simulink model "INDUCTION_ANALYSIS"  (R2022b)
settings: Solver=VariableStepAuto  StartTime=0.0  StopTime=0.5  RelTol=1e-3
libraries: simulink_extras x3, spsAsynchronousMachinepuUnitsLib x1, spsGroundLib x1, spsThreePhaseProgrammableVoltageSourceLib x1, spsThreePhaseVIMeasurementLib x1, spsThreePhaseBreakerLib x1, spsThreePhaseFaultLib x1, sps_lib x1
settings Model: Creator=ADA  LastModifiedBy=ADA
settings DebuggingCC: ParameterOverflowMsg=none  ParameterUnderflowMsg=error

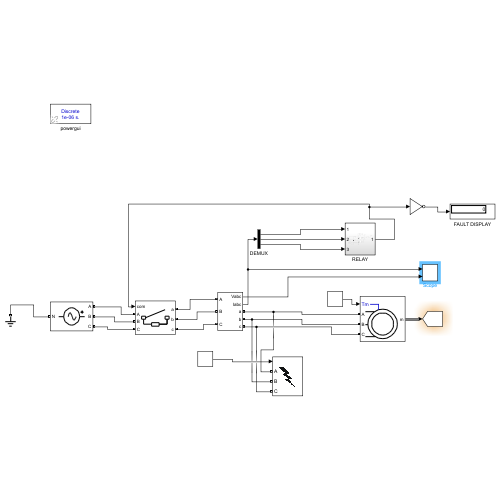
[thumbnail: Simulink's stored preview of the top-level diagram]
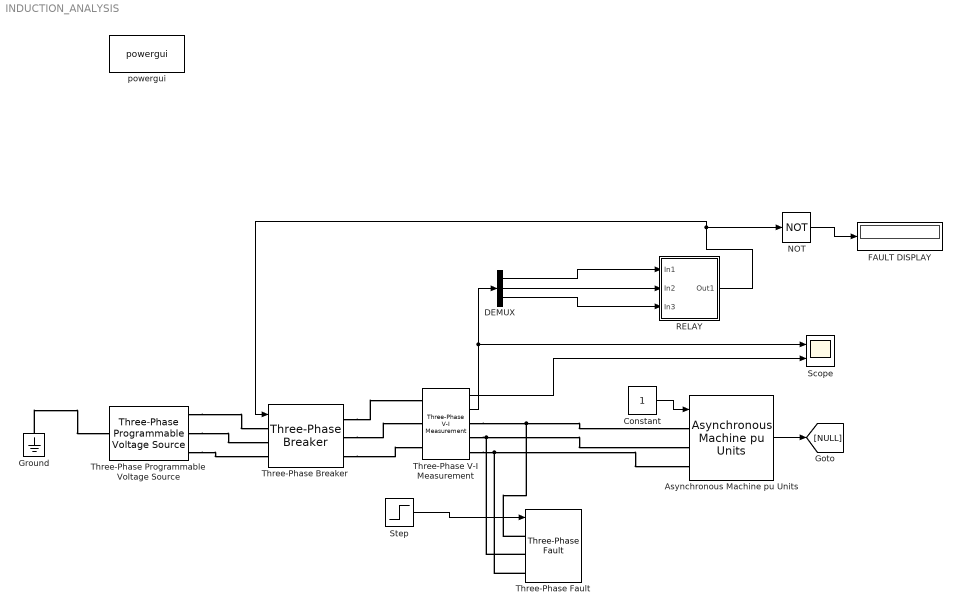
== system INDUCTION_ANALYSIS ==
  Asynchronous Machine pu Units : spsAsynchronousMachinepuUnitsLib/Asynchronous Machine pu Units  RotorType=Squirrel-cage  PresetModel=No  MechanicalLoad=Torque Tm  ShowDetailedParameters=on  ReferenceFrame=Rotor  Units=pu  MeasurementBus=off  NominalParameters=[3730 460 60]  VoltageRatio=1  Stator=[0.01965 0.0397]  Rotor=[0.01909 0.0397]  Cage1=[0.01909 0.0397]  Cage2=[0.01909 0.0397]  Lm=1.354  Mechanical=[0.09526 0.05479 2]  PolePairs=2  InitialConditions="[ 1,0   0,0,0   0,0,0 ]"  SimulateSaturation=off  Saturation="[0.212,0.4201,0.8125,1.0979,1.4799,2.2457,3.2586,4.5763,6.4763 ;   0.5,0.7,0.9,1,1.1,1.2 ,1.3,1.4,1.5]"  LoadFlowParameters=0  TsPowergui=0  TsBlock=-1  IterativeModel=Trapezoidal non iterative  IterativeDiscreteModel=Trapezoidal non iterative  Pmec=0
      settings: LibrarySourceBlock=|
      | sps_lib/Electrical Machines/Asynchronous Machine
      | pu Units
  Constant : Constant
  DEMUX : Demux  Outputs=3
  FAULT DISPLAY : Display
  Ground : spsGroundLib/Ground  LConnTagsString=a
  NOT : Logic  Operator=NOT  IconShape=distinctive  AllPortsSameDT=off  OutDataTypeStr=boolean
  RELAY : Subsystem
  Scope : Scope  NumInputPorts=2
  Step : Step  SampleTime=0
  Three-Phase Programmable Voltage Source : spsThreePhaseProgrammableVoltageSourceLib/Three-Phase Programmable Voltage Source  PositiveSequence="[100  0 50]"  VariationEntity=None  VariationType=Table of time-amplitude pairs  VariationTypeAlt=Step  VariationStep=0.5  VariationRate=10  VariationMagnitude=0.3  VariationFrequency=2  VariationTiming=[1 2]  VariationPhaseA=off  Amplitudes=[1 0.8 1.2 1.0]  TimeValues=[0 0.1 0.15 0.2]  HarmonicGeneration=off  HarmonicA=[3 0.2 -25 0]  HarmonicB=[2 0.15 35 2]  Timing="[0.05  3]"  BusType=swing  Pref=0  Qref=0  Qmin=-inf  Qmax=inf
  Three-Phase V-I Measurement : spsThreePhaseVIMeasurementLib/Three-Phase V-I Measurement  VoltageMeasurement=phase-to-ground  SetLabelV=off  LabelV=Vabc  Vpu=off  VpuLL=off  CurrentMeasurement=yes  SetLabelI=off  LabelI=Iabc  Ipu=off  Pbase=100e6  Vbase=500e3  OutputType=Complex  PhasorSimulation=off  PSBequivalent=0
  Three-Phase Breaker : spsThreePhaseBreakerLib/Three-Phase Breaker  InitialState=open  SwitchA=on  SwitchB=on  SwitchC=on  SwitchTimes="[1/60  5/60]"  External=on  BreakerResistance=0.01  SnubberResistance=1e6  SnubberCapacitance=inf  Measurements=None
  Three-Phase Fault : spsThreePhaseFaultLib/Three-Phase Fault  InitialStates=0  FaultA=on  FaultB=on  FaultC=on  GroundFault=on  SwitchTimes="[1/60  5/60]"  External=on  SwitchStatus=NaN  FaultResistance=0.001  GroundResistance=0.01  SnubberResistance=1e6  SnubberCapacitance=inf  Measurements=None
  powergui : sps_lib/powergui  Priority=1  SimulationMode=Discrete  SampleTime=1e-06  frequency=60  Iterations=50  frequencyindice=60  Pbase=100e6  ErrMax=1e-4  UnitsV=kV  UnitsW=MW  buscounter=0  FunctionMessages=off  echomessages=off  EnableUseOfTLC=off  CurrentSourceSwitches=off  DisableSnubberDevices=off  DisableRonSwitches=off  DisableVfSwitches=off  DisplayEquations=off  AutomaticDiscreteSolvers=off  SolverType=Tustin/Backward Euler (TBE)  Interpol=off  ExternalGateDelay=off  methode=off  Ts=100  x0status=blocks  SPID=on  SwTol=0  HookPort=off  NonlinearTolerance=1e-4  nMaxIteration=100  ContinueOnMaxIteration=off  RestoreLinks=warning  ResistiveCurrentMeasurement=off  Frange=[0:2:500]  Ylog=off  Xlog=on  ShowGrid=off  save=off  variable=ZData  structure=0  ZoomFFT=off  StartTime=0.0  cycles=1  DisplayStyle=1  fundamental=60  FreqAxis=off  MaxFrequency=1000  frequencyindicesteady=1  RmsSteady=1  display=off
  wires:
  Constant/1 -> Asynchronous Machine pu Units/1
  Three-Phase V-I Measurement/1 -> Scope/2
  Three-Phase V-I Measurement/2 -> DEMUX/1, Scope/1
  DEMUX/1 -> RELAY/1(In1)
  DEMUX/2 -> RELAY/2(In2)
  DEMUX/3 -> RELAY/3(In3)
  NOT/1 -> FAULT DISPLAY/1
  RELAY/1(Out1) -> Three-Phase Breaker/1, NOT/1
  Step/1 -> Three-Phase Fault/1
  Asynchronous Machine pu Units/1 -> [NULL]
  connections:
  Three-Phase Breaker/RConn1 -- Three-Phase V-I Measurement/LConn1
  Three-Phase Breaker/RConn2 -- Three-Phase V-I Measurement/LConn2
  Three-Phase Breaker/RConn3 -- Three-Phase V-I Measurement/LConn3
  Three-Phase Programmable Voltage Source/RConn1 -- Three-Phase Breaker/LConn1
  Three-Phase Programmable Voltage Source/RConn2 -- Three-Phase Breaker/LConn2
  Three-Phase Programmable Voltage Source/RConn3 -- Three-Phase Breaker/LConn3
  Ground/LConn1 -- Three-Phase Programmable Voltage Source/LConn1
  Three-Phase V-I Measurement/RConn1 -- Three-Phase Fault/LConn1 -- Asynchronous Machine pu Units/LConn1
  Three-Phase V-I Measurement/RConn2 -- Asynchronous Machine pu Units/LConn2 -- Three-Phase Fault/LConn2
  Three-Phase V-I Measurement/RConn3 -- Asynchronous Machine pu Units/LConn3 -- Three-Phase Fault/LConn3

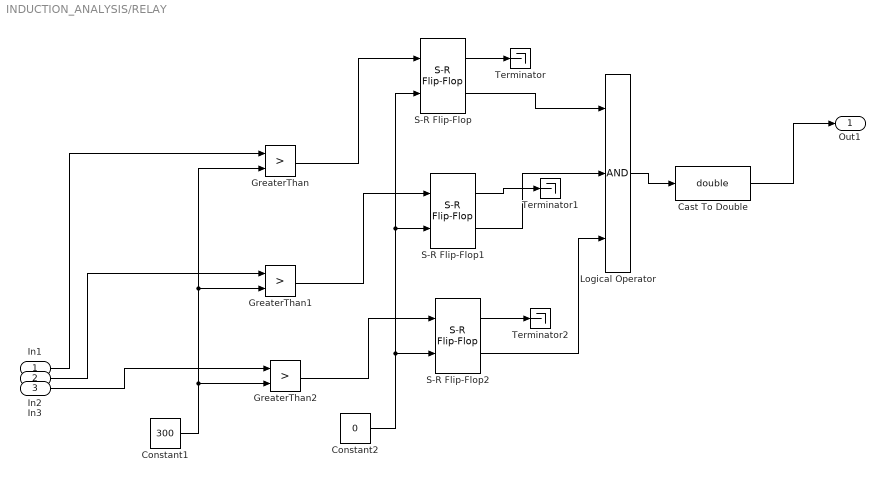
== system INDUCTION_ANALYSIS/RELAY ==
  In1 : Inport
  In2 : Inport  Port=2
  In3 : Inport  Port=3
  Cast To Double : DataTypeConversion  OutDataTypeStr=double  SaturateOnIntegerOverflow=off  RndMeth=Floor
  Constant1 : Constant  Value=300
  Constant2 : Constant  Value=0  OutDataTypeStr=boolean
  GreaterThan : RelationalOperator  Operator=>  OutDataTypeStr=boolean  RndMeth=Simplest  InputSameDT=off
  GreaterThan1 : RelationalOperator  Operator=>  OutDataTypeStr=boolean  RndMeth=Simplest  InputSameDT=off
  GreaterThan2 : RelationalOperator  Operator=>  OutDataTypeStr=boolean  RndMeth=Simplest  InputSameDT=off
  Logical Operator : Logic  Inputs=3  AllPortsSameDT=off  OutDataTypeStr=boolean
  S-R Flip-Flop : simulink_extras/Flip Flops/S-R Flip-Flop  initial_condition=0
  S-R Flip-Flop1 : simulink_extras/Flip Flops/S-R Flip-Flop  initial_condition=0
  S-R Flip-Flop2 : simulink_extras/Flip Flops/S-R Flip-Flop  initial_condition=0
  Terminator : Terminator
  Terminator1 : Terminator
  Terminator2 : Terminator
  Out1 : Outport
  wires:
  Constant2/1 -> S-R Flip-Flop2/2, S-R Flip-Flop1/2, S-R Flip-Flop/2
  Logical Operator/1 -> Cast To Double/1
  Constant1/1 -> GreaterThan1/2, GreaterThan/2, GreaterThan2/2
  S-R Flip-Flop2/2 -> Logical Operator/3
  S-R Flip-Flop/1 -> Terminator/1
  S-R Flip-Flop1/1 -> Terminator1/1
  GreaterThan1/1 -> S-R Flip-Flop1/1
  S-R Flip-Flop2/1 -> Terminator2/1
  GreaterThan/1 -> S-R Flip-Flop/1
  GreaterThan2/1 -> S-R Flip-Flop2/1
  S-R Flip-Flop/2 -> Logical Operator/1
  S-R Flip-Flop1/2 -> Logical Operator/2
  In2/1 -> GreaterThan1/1
  In1/1 -> GreaterThan/1
  In3/1 -> GreaterThan2/1
  Cast To Double/1 -> Out1/1
